simulink model "AutoMotiveSuspension0108"  (R2025a)
settings: Solver=VariableStepAuto  StartTime=0.0  StopTime=10.0  RelTol=1e-3
InitFcn:
  | param_setup
StopFcn:
  | if exist('sldemo_suspn_output')
  | sldemo_suspgraph
  | end
undefined symbols (not defined in the file): cf, cr, Iyy, kf, kr, Lf, Lr, Mb
CloseFcn:
  | f exist('suspnFigH')
  | 
  | if ishghandle(suspnFigH,'figure')
  | 
  | close(suspnFigH)
  | 
  | end
  | 
  | clear suspnFigH
  | 
  | end
  | 
  | if exist('suspnAxH'), clear suspnAxH; end
settings Model: Creator=sanghoon  LastModifiedBy=sanghoon
settings DataIOCC: SignalLoggingName=sldemo_suspn_output

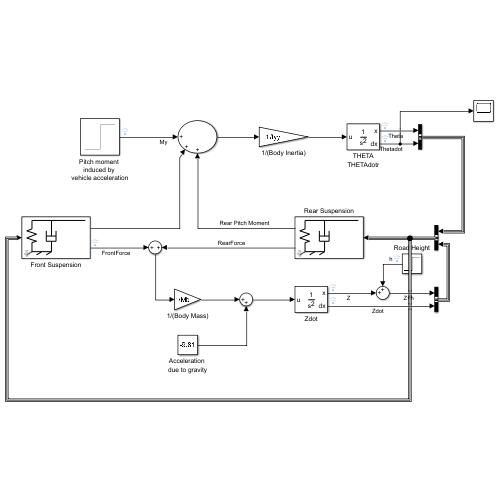
[thumbnail: Simulink's stored preview of the top-level diagram]
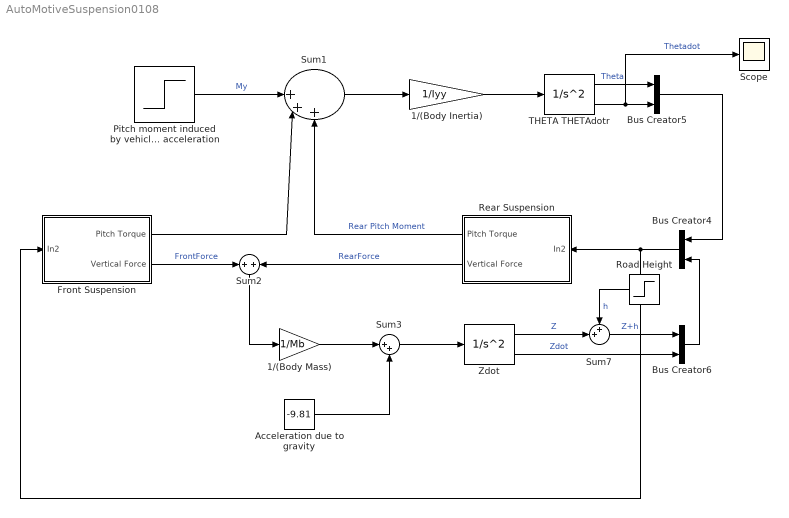
== system AutoMotiveSuspension0108 ==
  1/(Body Inertia) : Gain  Gain=1/Iyy
  1/(Body Mass) : Gain  Gain=1/Mb
  Acceleration due to gravity : Constant  Value=-9.81
  Bus Creator4 : BusCreator  Inputs=2
  Bus Creator5 : BusCreator  Inputs=2
  Bus Creator6 : BusCreator  Inputs=2
  Front Suspension : Subsystem  mask{K=kf, C=cf, L=-Lf}
      mask prompts: K "Stiffness = spring rate:"; C "Damping rate:"; L "Moment arm:"
      mask DialogControl ParameterGroupVar Prompt: 파라미터
      mask Display: plot(-1, 0, 13, 12, [1 12], [11 11], [1 5], [2 2], [1 2], [4.5 5], [2 0], [5 6], [0 2], [6 7], [2 0], [7 8], [0 1], [8 8.5], [1 1], [8.5 11], [1 1], [2 4.5], [5 5], [2 5], [4 6], [5 5], [4 4], [5 8], [6 6], [5 8], [4 6], [6.5 6.5], [5 5], [6.5 11], [0 1], [1 2], [2 3], [1 2], [4 5], [1 2])
  Pitch moment induced by vehicle acceleration : Step  Time=3  After=100  SampleTime=0
  Rear Suspension : Subsystem  mask{K=kr, C=cr, L=Lr}
      mask prompts: K "Stiffness = spring rate:"; C "Damping rate:"; L "Moment arm:"
      mask DialogControl ParameterGroupVar Prompt: 파라미터
      mask Display: plot(-1, 0, 13, 12, [1 12], [11 11], [1 5], [2 2], [1 2], [4.5 5], [2 0], [5 6], [0 2], [6 7], [2 0], [7 8], [0 1], [8 8.5], [1 1], [8.5 11], [1 1], [2 4.5], [5 5], [2 5], [4 6], [5 5], [4 4], [5 8], [6 6], [5 8], [4 6], [6.5 6.5], [5 5], [6.5 11], [0 1], [1 2], [2 3], [1 2], [4 5], [1 2])
  Road Height : Step  Time=7  After=0.01  SampleTime=0
  Scope : Scope
      settings: ActiveDisplayYMinimum=-1  ActiveDisplayYMaximum=1
  Sum1 : Sum  Inputs=||+++
  Sum2 : Sum
  Sum3 : Sum  Inputs=|++
  Sum7 : Sum  Inputs=++|
  THETA THETAdotr : SecondOrderIntegrator  ICX=-8.7e-20  ICDXDT=8.04e-28
  Zdot : SecondOrderIntegrator  ICX=-0.12
  wires:
  Pitch moment induced by vehicle acceleration/1 -> Sum1/1  "My"
  Sum1/1 -> 1/(Body Inertia)/1
  Bus Creator4/1 -> Front Suspension/1(In2), Rear Suspension/1(In2)
  1/(Body Inertia)/1 -> THETA THETAdotr/1
  Sum2/1 -> 1/(Body Mass)/1
  Bus Creator6/1 -> Bus Creator4/2
  1/(Body Mass)/1 -> Sum3/1
  Zdot/2 -> Bus Creator6/2  "Zdot"
  Sum3/1 -> Zdot/1
  Bus Creator5/1 -> Bus Creator4/1
  THETA THETAdotr/2 -> Scope/1, Bus Creator5/2  "Thetadot"
  Rear Suspension/1(Pitch Torque) -> Sum1/3  "Rear Pitch Moment"
  THETA THETAdotr/1 -> Bus Creator5/1  "Theta"
  Sum7/1 -> Bus Creator6/1  "Z+h"
  Road Height/1 -> Sum7/1  "h"
  Front Suspension/1(Pitch Torque) -> Sum1/2
  Zdot/1 -> Sum7/2  "Z"
  Acceleration due to gravity/1 -> Sum3/2
  Rear Suspension/2(Vertical Force) -> Sum2/2  "RearForce"
  Front Suspension/2(Vertical Force) -> Sum2/1  "FrontForce"

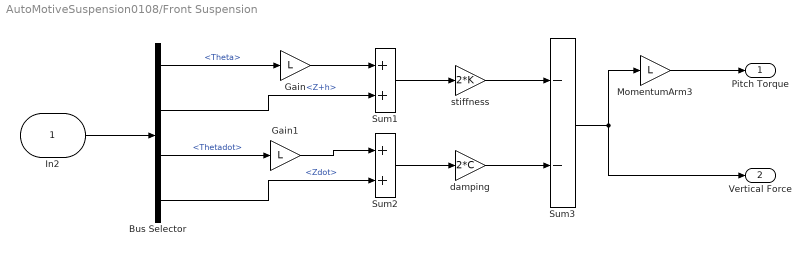
== system AutoMotiveSuspension0108/Front Suspension ==
  In2 : Inport
  Bus Selector : BusSelector  OutputSignals=signal1.Theta,signal2.Z+h,signal1.Thetadot,signal2.Zdot
  Gain : Gain  Gain=L
  Gain1 : Gain  Gain=L
  MomentumArm3 : Gain  Gain=L
  Sum1 : Sum
  Sum2 : Sum
  Sum3 : Sum  Inputs=--
  damping : Gain  Gain=2*C
  stiffness : Gain  Gain=2*K
  Pitch Torque : Outport
  Vertical Force : Outport  Port=2
  wires:
  Sum1/1 -> stiffness/1
  Sum3/1 -> Vertical Force/1, MomentumArm3/1
  damping/1 -> Sum3/2
  stiffness/1 -> Sum3/1
  MomentumArm3/1 -> Pitch Torque/1
  Sum2/1 -> damping/1
  Gain/1 -> Sum1/1
  Gain1/1 -> Sum2/1
  In2/1 -> Bus Selector/1
  Bus Selector/1 -> Gain/1  "<Theta>"
  Bus Selector/2 -> Sum1/2  "<Z+h>"
  Bus Selector/3 -> Gain1/1  "<Thetadot>"
  Bus Selector/4 -> Sum2/2  "<Zdot>"

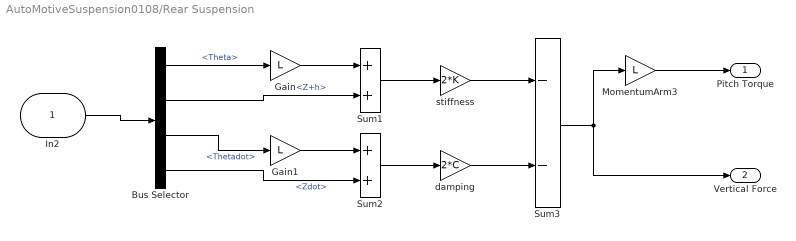
== system AutoMotiveSuspension0108/Rear Suspension ==
  In2 : Inport
  Bus Selector : BusSelector  OutputSignals=signal1.Theta,signal2.Z+h,signal1.Thetadot,signal2.Zdot
  Gain : Gain  Gain=L
  Gain1 : Gain  Gain=L
  MomentumArm3 : Gain  Gain=L
  Sum1 : Sum
  Sum2 : Sum
  Sum3 : Sum  Inputs=--
  damping : Gain  Gain=2*C
  stiffness : Gain  Gain=2*K
  Pitch Torque : Outport
  Vertical Force : Outport  Port=2
  wires:
  Sum1/1 -> stiffness/1
  Sum3/1 -> Vertical Force/1, MomentumArm3/1
  damping/1 -> Sum3/2
  stiffness/1 -> Sum3/1
  MomentumArm3/1 -> Pitch Torque/1
  Sum2/1 -> damping/1
  Gain/1 -> Sum1/1
  Gain1/1 -> Sum2/1
  In2/1 -> Bus Selector/1
  Bus Selector/1 -> Gain/1  "<Theta>"
  Bus Selector/2 -> Sum1/2  "<Z+h>"
  Bus Selector/3 -> Gain1/1  "<Thetadot>"
  Bus Selector/4 -> Sum2/2  "<Zdot>"
